simulink model "ModelF"  (R2025b)
settings: Solver=VariableStepAuto  StartTime=0.0  StopTime=1800  RelTol=1e-3
values from neighbouring files (symbols this model uses):
  Af = 2.46    [MainF.m]
  Cd = Input_Parameters(i,2)    [MainF.m]
  ego_length = 4    [MainF.m]
  g = 9.81    [MainF.m]
  m = Input_Parameters(i,1)    [MainF.m]
  max_ac = 2    [MainF.m]
  min_ac = -3    [MainF.m]
  rho_air = 1.2256    [MainF.m]
  slope = Input_Parameters(i,5)    [MainF.m]
  standstill_distance = 1.5    [MainF.m]
  time_gap = Input_Parameters(i,3)    [MainF.m]
  v_des = Input_Parameters(i,6)    [MainF.m]
  v_ego = 1    [MainF.m]
  verr_gain = 0.5    [MainF.m]
  vx_gain = 0.6    [MainF.m]
  x_ego = 0    [MainF.m]
  x_leader = 30    [MainF.m]
  xerr_gain = 0.2    [MainF.m]
undefined symbols (not defined in the file or in its folder): magnitude
libraries: autolibshared x1
settings Model: Creator=Angelo  LastModifiedBy=r1504
settings OptimizationCC: ReuseModelBlockBuffer=off
settings RTWCC: GPUComputeCapability=3.5

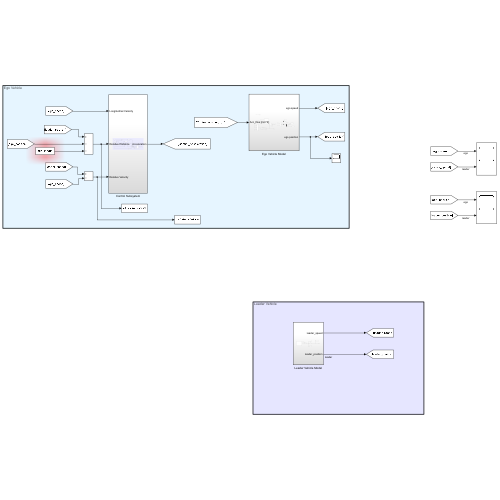
[thumbnail: Simulink's stored preview of the top-level diagram]
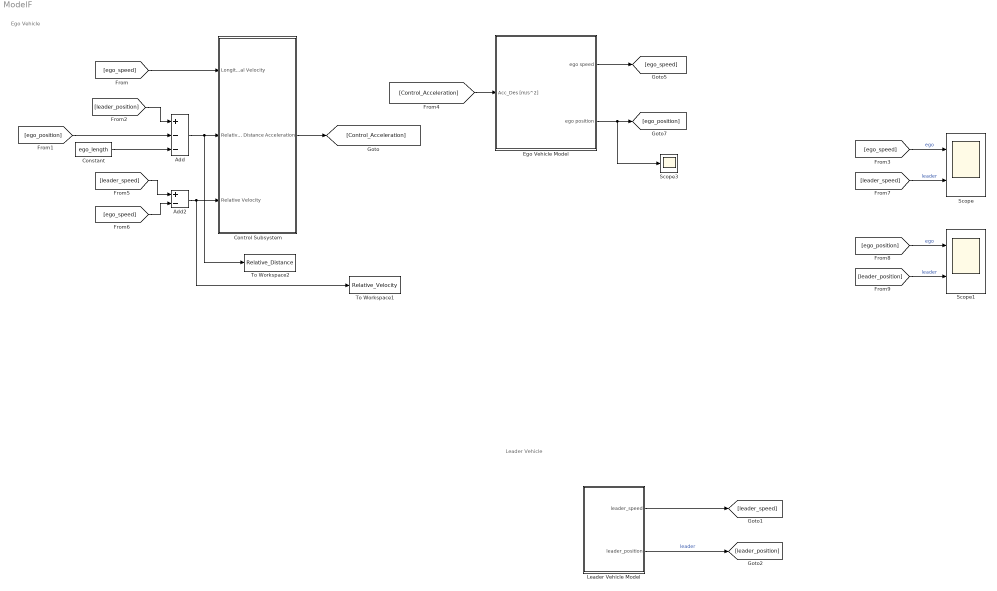
== system ModelF ==
  note: Ego Vehicle
  note: Leader Vehicle
  Add : Sum  Inputs=+--
  Add2 : Sum  Inputs=+-
  Constant : Constant  Value=ego_length
  Control Subsystem : Subsystem
  Ego Vehicle Model : Subsystem
  Leader Vehicle Model : Subsystem
  Scope : Scope  NumInputPorts=2
      settings: ActiveDisplayYMinimum=-0.065317862974867857  ActiveDisplayYMaximum=8.1260678814883782
  Scope1 : Scope  NumInputPorts=2
      settings: ActiveDisplayYMinimum=301.30874978128895  ActiveDisplayYMaximum=428.44171094881705  DataLoggingVariableName=ScopeData2
  Scope3 : Scope
      settings: ActiveDisplayYMinimum=-293.86381  ActiveDisplayYMaximum=2644.77431  DataLoggingVariableName=ScopeData3
  To Workspace1 : ToWorkspace  VariableName=Relative_Velocity  SampleTime=0.1
      settings: Save2DSignal=2-D array (concatenate along first dimension)
  To Workspace2 : ToWorkspace  VariableName=Relative_Distance  SampleTime=0.1
      settings: Save2DSignal=2-D array (concatenate along first dimension)
  wires:
  [Control_Acceleration] -> Ego Vehicle Model/1(Acc_Des [m/s^2])
  Ego Vehicle Model/1(ego speed) -> [ego_speed]
  Ego Vehicle Model/2(ego position) -> [ego_position], Scope3/1
  Control Subsystem/1(Acceleration) -> [Control_Acceleration]
  [ego_speed] -> Control Subsystem/1(Longitudinal Velocity)
  Leader Vehicle Model/2(leader_position) -> [leader_position]  "leader"
  Add/1 -> To Workspace2/1, Control Subsystem/2(Relative Distance)
  [leader_position] -> Add/1
  [ego_position] -> Add/2
  [ego_speed] -> Add2/2
  [leader_speed] -> Add2/1
  Add2/1 -> To Workspace1/1, Control Subsystem/3(Relative Velocity)
  [ego_speed] -> Scope/1  "ego"
  [leader_speed] -> Scope/2  "leader"
  [leader_position] -> Scope1/2  "leader"
  [ego_position] -> Scope1/1  "ego"
  Leader Vehicle Model/1(leader_speed) -> [leader_speed]
  Constant/1 -> Add/3

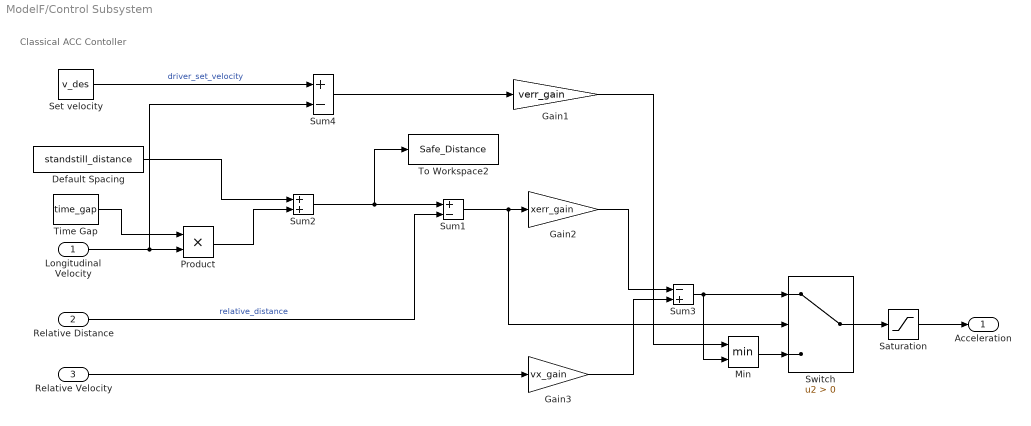
== system ModelF/Control Subsystem ==
  note: Classical ACC Contoller
  Longitudinal Velocity : Inport
  Relative Distance : Inport  Port=2
  Relative Velocity : Inport  Port=3
  Default Spacing : Constant  Value=standstill_distance  SampleTime=-1
  Gain1 : Gain  Gain=verr_gain
  Gain2 : Gain  Gain=xerr_gain
  Gain3 : Gain  Gain=vx_gain
  Min : MinMax  Inputs=2
  Product : Product
  Saturation : Saturate  UpperLimit=max_ac  LowerLimit=min_ac
  Set velocity : Constant  Value=v_des  SampleTime=-1
  Sum1 : Sum  Inputs=+-
  Sum2 : Sum
  Sum3 : Sum  Inputs=-+
  Sum4 : Sum  Inputs=+-
  Switch : Switch  Criteria=u2 > Threshold  SaturateOnIntegerOverflow=off  InputSameDT=off
  Time Gap : Constant  Value=time_gap  SampleTime=-1
  To Workspace2 : ToWorkspace  VariableName=Safe_Distance  SampleTime=0.1
      settings: Save2DSignal=2-D array (concatenate along first dimension)
  Acceleration : Outport  VectorParamsAs1DForOutWhenUnconnected=off
  wires:
  Product/1 -> Sum2/2
  Switch/1 -> Saturation/1
  Sum1/1 -> Switch/2, Gain2/1
  Default Spacing/1 -> Sum2/1
  Min/1 -> Switch/3
  Gain3/1 -> Sum3/2
  Set velocity/1 -> Sum4/1  "driver_set_velocity"
  Time Gap/1 -> Product/1
  Relative Velocity/1 -> Gain3/1
  Longitudinal Velocity/1 -> Product/2, Sum4/2
  Sum4/1 -> Gain1/1
  Saturation/1 -> Acceleration/1
  Relative Distance/1 -> Sum1/2  "relative_distance"
  Sum3/1 -> Min/2, Switch/1
  Gain1/1 -> Min/1
  Gain2/1 -> Sum3/1
  Sum2/1 -> To Workspace2/1, Sum1/1

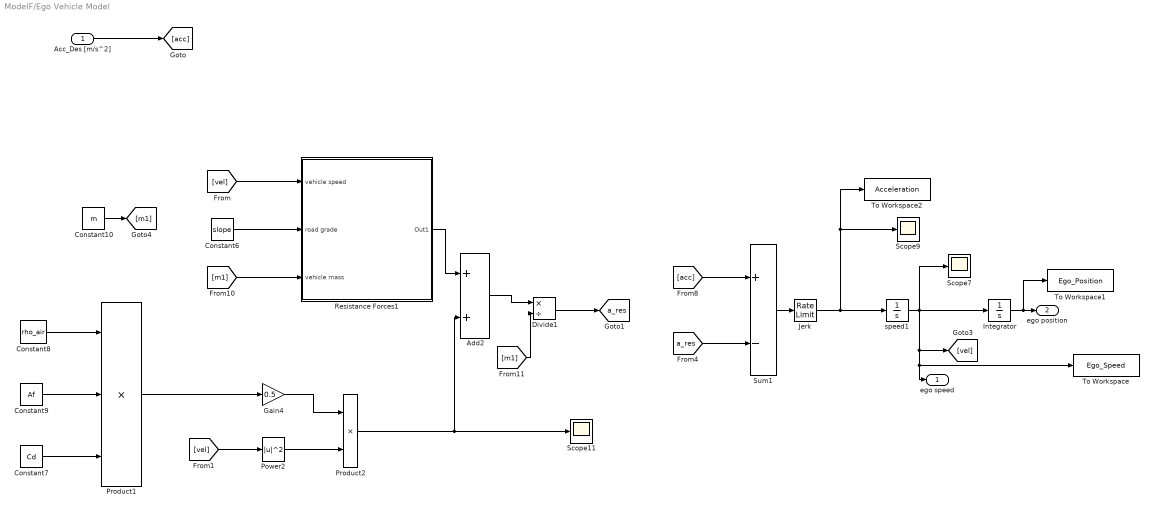
== system ModelF/Ego Vehicle Model ==
  Acc_Des [m/s^2] : Inport
  Add2 : Sum
  Constant10 : Constant  Value=m
  Constant6 : Constant  Value=slope
  Constant7 : Constant  Value=Cd
  Constant8 : Constant  Value=rho_air
  Constant9 : Constant  Value=Af
  Divide1 : Product  Inputs=*/
  Gain4 : Gain  Gain=0.5
  Integrator : Integrator  InitialCondition=x_ego
  Jerk : RateLimiter  RisingSlewLimit=15  FallingSlewLimit=-15
  Power2 : Math  Operator=magnitude^2  SignedPower=on
  Product1 : Product  Inputs=3
  Product2 : Product
  Resistance Forces1 : Subsystem
  Scope11 : Scope
      settings: ActiveDisplayYMinimum=185.1088  ActiveDisplayYMaximum=301.23834  DataLoggingVariableName=ScopeData5
  Scope7 : Scope
      settings: ActiveDisplayYMinimum=-2.3804  ActiveDisplayYMaximum=23.65152  DataLoggingVariableName=ScopeData6
  Scope9 : Scope
      settings: ActiveDisplayYMinimum=-2.03075  ActiveDisplayYMaximum=0.26409  DataLoggingVariableName=ScopeData8
  Sum1 : Sum  Inputs=+-
  To Workspace : ToWorkspace  VariableName=Ego_Speed  SampleTime=0.1
      settings: Save2DSignal=2-D array (concatenate along first dimension)
  To Workspace1 : ToWorkspace  VariableName=Ego_Position  SampleTime=0.1
      settings: Save2DSignal=2-D array (concatenate along first dimension)
  To Workspace2 : ToWorkspace  VariableName=Acceleration  SampleTime=0.1
      settings: Save2DSignal=2-D array (concatenate along first dimension)
  speed1 : Integrator  InitialCondition=v_ego  LimitOutput=on  UpperSaturationLimit=40  LowerSaturationLimit=0
  ego speed : Outport
  ego position : Outport  Port=2
  tag scope: a_res=global
  wires:
  Acc_Des [m/s^2]/1 -> [acc]
  Integrator/1 -> ego position/1, To Workspace1/1
  Resistance Forces1/1(Out1) -> Add2/1
  Product1/1 -> Gain4/1
  Constant8/1 -> Product1/1
  Jerk/1 -> To Workspace2/1, Scope9/1, speed1/1
  [m1] -> Resistance Forces1/3(vehicle mass)
  Constant9/1 -> Product1/2
  Constant10/1 -> [m1]
  [m1] -> Divide1/2
  Constant7/1 -> Product1/3
  Divide1/1 -> [a_res]
  Add2/1 -> Divide1/1
  Product2/1 -> Scope11/1, Add2/2
  speed1/1 -> Scope7/1, [vel], To Workspace/1, ego speed/1, Integrator/1
  [vel] -> Resistance Forces1/1(vehicle speed)
  Power2/1 -> Product2/2
  Sum1/1 -> Jerk/1
  [acc] -> Sum1/1
  [vel] -> Power2/1
  Gain4/1 -> Product2/1
  Constant6/1 -> Resistance Forces1/2(road grade)
  [a_res] -> Sum1/2

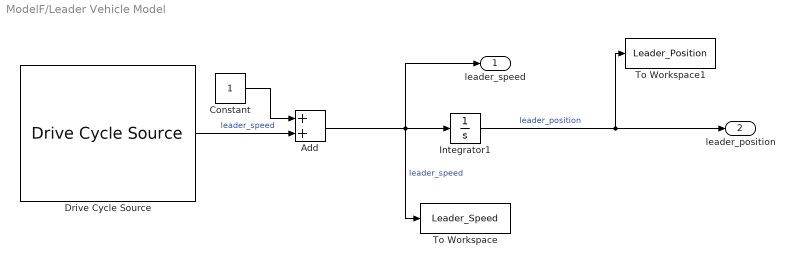
== system ModelF/Leader Vehicle Model ==
  Add : Sum
  Constant : Constant
  Drive Cycle Source : autolibshared/Drive Cycle Source  cycleVar=WLTP Class 3  fileVar=cycleFTP75.mat  tfinal="1800  seconds"  cycleRepeat=off  outAccPort=off  outGearPort=off  gearList=No gear data  t_wot1=5  xdot_woto=0  xdot_wot1=30  t_wot2=20  xdot_wot2=0  t_wotend=30  srcUnit=m/s  outUnit=m/s  srcAccUnit=m/s/s  outAccUnit=m/s^2  dt=0  aMode=1  faultOption=off  velBnd=2  velBndUnit=mph  inUnit=m/s  timeBnd=1  failOption=off  stopSim=off  maxFaultCnt=10  maxFaultTime=2  maxTotFaultTime=15  traceOption=off  dtTrace=1  traceWindow=10  lastDCname=WLTP Class 3  lastOutUnit=mph  lastDT=0  lastTB=1  lastSB=2  forceCalcBound=off
  Integrator1 : Integrator  InitialCondition=x_leader
  To Workspace : ToWorkspace  VariableName=Leader_Speed  SampleTime=0.1
      settings: Save2DSignal=2-D array (concatenate along first dimension)
  To Workspace1 : ToWorkspace  VariableName=Leader_Position  SampleTime=0.1
      settings: Save2DSignal=2-D array (concatenate along first dimension)
  leader_speed : Outport
  leader_position : Outport  Port=2
  wires:
  Integrator1/1 -> To Workspace1/1, leader_position/1  "leader_position"
  Add/1 -> To Workspace/1, leader_speed/1, Integrator1/1  "leader_speed"
  Drive Cycle Source/1 -> Add/2  "leader_speed"
  Constant/1 -> Add/1

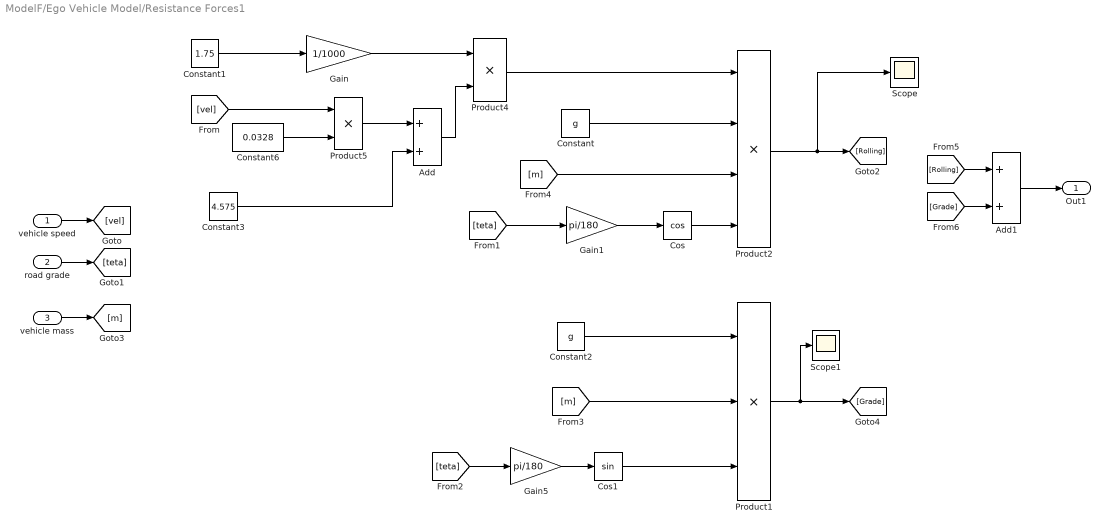
== system ModelF/Ego Vehicle Model/Resistance Forces1 ==
  vehicle speed : Inport
  road grade : Inport  Port=2
  vehicle mass : Inport  Port=3
  Add : Sum
  Add1 : Sum
  Constant : Constant  Value=g
  Constant1 : Constant  Value=1.75
  Constant2 : Constant  Value=g
  Constant3 : Constant  Value=4.575
  Constant6 : Constant  Value=0.0328
  Cos : Trigonometry  Operator=cos
  Cos1 : Trigonometry
  Gain : Gain  Gain=1/1000
  Gain1 : Gain  Gain=pi/180
  Gain5 : Gain  Gain=pi/180
  Product1 : Product  Inputs=3
  Product2 : Product  Inputs=4
  Product4 : Product
  Product5 : Product
  Scope : Scope
      settings: ActiveDisplayYMinimum=129.19596  ActiveDisplayYMaximum=132.03061  DataLoggingVariableName=ScopeData4
  Scope1 : Scope
      settings: ActiveDisplayYMinimum=-1  ActiveDisplayYMaximum=1  DataLoggingVariableName=ScopeData5
  Out1 : Outport
  wires:
  Constant6/1 -> Product5/2
  Add/1 -> Product4/2
  Constant3/1 -> Add/2
  Gain/1 -> Product4/1
  Constant/1 -> Product2/2
  Product4/1 -> Product2/1
  Product5/1 -> Add/1
  [vel] -> Product5/1
  vehicle speed/1 -> [vel]
  Product2/1 -> Scope/1, [Rolling]
  [m] -> Product2/3
  Cos/1 -> Product2/4
  road grade/1 -> [teta]
  [teta] -> Gain1/1
  [teta] -> Gain5/1
  Cos1/1 -> Product1/3
  [m] -> Product1/2
  Product1/1 -> Scope1/1, [Grade]
  Constant2/1 -> Product1/1
  vehicle mass/1 -> [m]
  Add1/1 -> Out1/1
  [Rolling] -> Add1/1
  [Grade] -> Add1/2
  Gain5/1 -> Cos1/1
  Gain1/1 -> Cos/1
  Constant1/1 -> Gain/1
